simulink subsystem "CyclesFromSeconds"  (R2020b)
settings: Solver=VariableStepAuto  StartTime=0.0  StopTime=10.0  RelTol=1e-3
model mask{sec=0}
  mask prompts: sec "Seconds to convert to cycles"
values from neighbouring files (symbols this model uses):
  tc = Constants{10}    [Load_config.m]
settings Model: Creator=Marcus  LastModifiedBy=Marcus

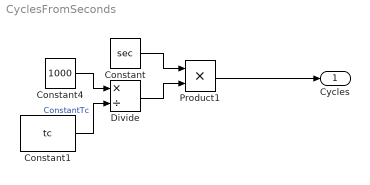
== system CyclesFromSeconds ==
  Constant : Constant  Value=sec
  Constant1 : Constant  Value=tc
  Constant4 : Constant  Value=1000
  Divide : Product  Inputs=*/
  Product1 : Product  OutDataTypeStr=int32  RndMeth=Ceiling
  Cycles : Outport
  wires:
  Constant4/1 -> Divide/1
  Product1/1 -> Cycles/1
  Constant/1 -> Product1/1
  Constant1/1 -> Divide/2  "ConstantTc"
  Divide/1 -> Product1/2
